simulink model "controller1"  (R2021b)
settings: Solver=ode45  StartTime=0.0  StopTime=10.0  RelTol=1e-3
libraries: cstblocks x2
settings Model: Creator=dabner  LastModifiedBy=dabner

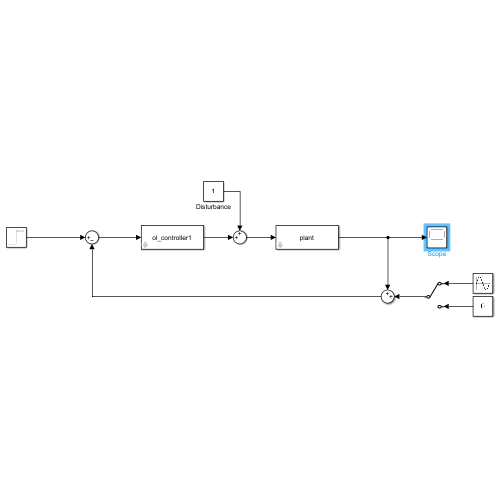
[thumbnail: Simulink's stored preview of the top-level diagram]
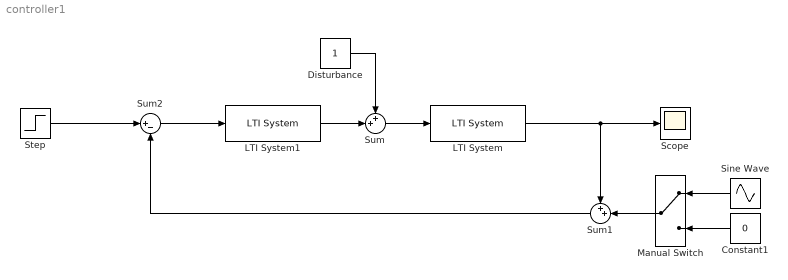
== system controller1 ==
  Constant1 : Constant  Value=0
  Disturbance : Constant
  LTI System : cstblocks/LTI System  sys=plant  IC=[]
  LTI System1 : cstblocks/LTI System  sys=ol_controller1  IC=[]
  Manual Switch : ManualSwitch
  Scope : Scope
  Sine Wave : Sin  Frequency=20  SampleTime=0
  Step : Step  SampleTime=0
  Sum : Sum  Inputs=++|
  Sum1 : Sum  Inputs=++|
  Sum2 : Sum  Inputs=|+-
  wires:
  LTI System/1 -> Sum1/1, Scope/1
  Step/1 -> Sum2/1
  Sum2/1 -> LTI System1/1
  LTI System1/1 -> Sum/2
  Sum/1 -> LTI System/1
  Sum1/1 -> Sum2/2
  Disturbance/1 -> Sum/1
  Manual Switch/1 -> Sum1/2
  Sine Wave/1 -> Manual Switch/1
  Constant1/1 -> Manual Switch/2
